simulink model "proyectoscada"  (R2016b)
settings: Solver=ode1  StartTime=0.0  StopTime=inf  FixedStep=50e-6  RelTol=1e-3
libraries: powerlib x17, rtlab x15, powerlib_meascontrol x10, sps_avr x1
settings Model: Creator=Estudiante  LastModifiedBy=Laboratorio

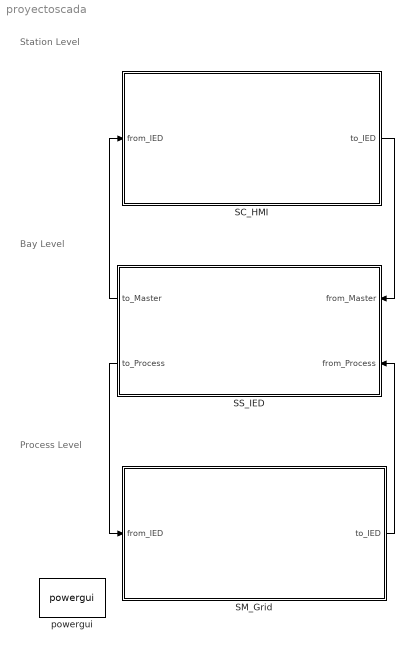
== system proyectoscada ==
  note: Station Level
  note: Bay Level
  note: Process Level
  SC_HMI : Subsystem
  SM_Grid : Subsystem
  SS_IED : Subsystem
  powergui : powerlib/powergui  Priority=1  SimulationMode=Discrete  SolverType=Backward Euler  SampleTime=50e-6  frequency=60  SPID=off  DisableSnubberDevices=off  DisableRonSwitches=off  DisableVfSwitches=off  SwTol=0  DisplayEquations=off  Interpol=off  ExternalGateDelay=off  methode=off  Ts=10  FunctionMessages=off  echomessages=off  HookPort=off  EnableUseOfTLC=off  x0status=blocks  frequencyindice=60  Pbase=100e6  ErrMax=1e-4  Iterations=50  UnitsV=kV  UnitsW=MW  buscounter=0  RestoreLinks=warning  ResistiveCurrentMeasurement=off  Frange=[0:2:500]  Ylog=off  Xlog=on  ShowGrid=off  save=off  variable=ZData  structure=0  ZoomFFT=off  StartTime=0.0  cycles=1  DisplayStyle=1  fundamental=60  FreqAxis=off  MaxFrequency=1000  frequencyindicesteady=1  RmsSteady=1  display=off
  wires:
  SS_IED/2(to_Process) -> SM_Grid/1(from_IED)
  SM_Grid/1(to_IED) -> SS_IED/2(from_Process)
  SC_HMI/1(to_IED) -> SS_IED/1(from_Master)
  SS_IED/1(to_Master) -> SC_HMI/1(from_IED)

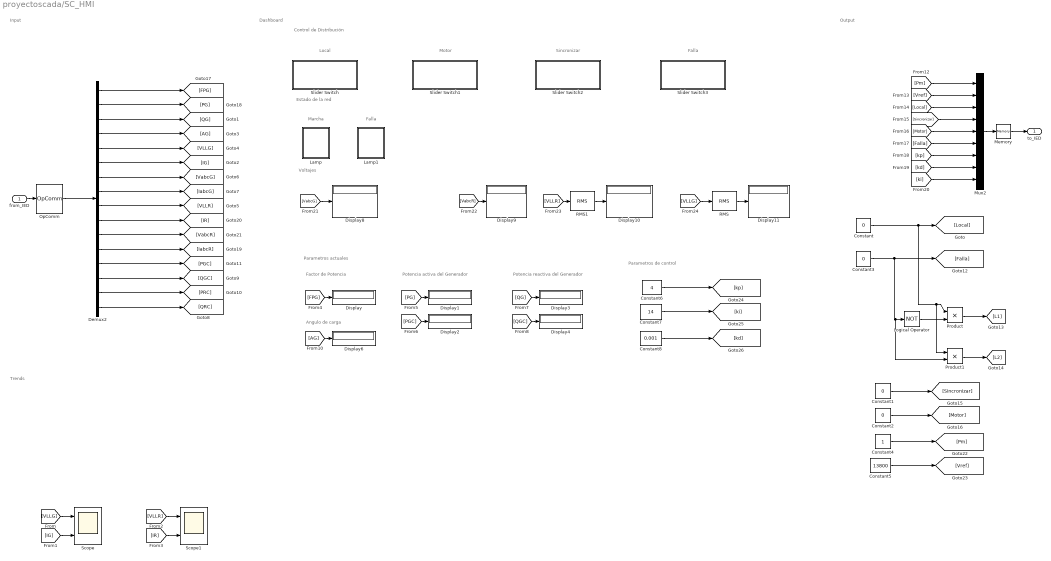
== system proyectoscada/SC_HMI ==
  note: Dashboard
  note: Input
  note: Factor de Potencia
  note: Falla
  note: Marcha
  note: Control de Distribución
  note: Falla
  note: Motor
  note: Sincronizar
  note: Local
  note: Estado de la red
  note: Voltajes
  note: Parametros actuales
  note: Potencia activa del Generador
  note: Potencia reactiva del Generador
  note: Angulo de carga
  note: Trends
  note: Output
  note: Parametros de control
  from_IED : Inport
  Constant{,1..3} (4 alike) : Constant  Value=0
  Constant4 : Constant
  Constant5 : Constant  Value=13800
  Constant6 : Constant  Value=4
  Constant7 : Constant  Value=14
  Constant8 : Constant  Value=0.001
  Demux2 : Demux  Outputs=[1 1 1 1 1 1 3 3 1 1 3 3 1 1 1 1]
  Display{,1..4,6,8..11} (10 alike) : Display
  Lamp : Subsystem  DialogController=hmiCreateDDGDialog  IsWebBlock=on  mask(MWDashboardBlock){webBlockId=f6681ff5-1f51-4868-82b0-294eaddaf335, webBlockType=lamp, ShowInLibBrowser=on, ShowInitialText=on, HMISrcModelName=proyectoscada}
      mask prompts: webBlockType "WebBlock Type"; HMISrcModelName "Source Model"
      mask help: SimulinkHMI:dialogs:LampDialogDesc
      mask Help: helpview([docroot '/mapfiles/simulink.map'], 'hmi_lamp')
      mask Display:
      | if strcmp(get_param(bdroot(gcb),'BlockDiagramType'), 'library')
      |     image([(matlabroot) '/toolbox/simulink/hmi/icons/Lamp.png']);
      | end
  Lamp1 : Subsystem  DialogController=hmiCreateDDGDialog  IsWebBlock=on  mask(MWDashboardBlock){webBlockId=feaf209c-0dec-4196-b8e9-5f0cb4ab0a6e, webBlockType=lamp, ShowInLibBrowser=on, ShowInitialText=on, HMISrcModelName=proyectoscada}
      mask prompts: webBlockType "WebBlock Type"; HMISrcModelName "Source Model"
      mask help: SimulinkHMI:dialogs:LampDialogDesc
      mask Help: helpview([docroot '/mapfiles/simulink.map'], 'hmi_lamp')
      mask Display:
      | if strcmp(get_param(bdroot(gcb),'BlockDiagramType'), 'library')
      |     image([(matlabroot) '/toolbox/simulink/hmi/icons/Lamp.png']);
      | end
  Logical Operator : Logic  Operator=NOT  AllPortsSameDT=off  OutDataTypeStr=boolean
  Memory : Memory
  Mux2 : Mux  Inputs=9
  OpComm : rtlab/OpComm  nbport=1  groupe_acq=1  subsys_rate=0  st=0  Synchronization=on  Interpolation=on  Threshold=1.0  Missed_Data=off  Sim_Time=off  Samples=off  dynSigOut=off  from_console=0  warning_done=off  writeOpCommFile=off  Offset=off
  Product : Product
  Product1 : Product
  RMS : powerlib_meascontrol/Measurements/RMS  TrueRMS=on  Freq=60  RMSInit=120  Ts=0
  RMS1 : powerlib_meascontrol/Measurements/RMS  TrueRMS=on  Freq=60  RMSInit=120  Ts=0
  Scope : Scope  NumInputPorts=2
  Scope1 : Scope  NumInputPorts=2
  Slider Switch : Subsystem  DialogController=hmiCreateDDGDialog  IsWebBlock=on  mask(MWDashboardBlock){webBlockId=af04694c-61e9-4dac-be57-759f0575d0dc, webBlockType=sliderswitch, ShowInLibBrowser=on, ShowInitialText=on, HMISrcModelName=proyectoscada}
      mask prompts: webBlockId "WebBlock Id"; webBlockType "WebBlock Type"; HMISrcModelName "Source Model"
      mask help: SimulinkHMI:dialogs:SwitchDialogDesc
      mask Help: helpview([docroot '/mapfiles/simulink.map'], 'hmi_slider_switch')
      mask Display:
      | if strcmp(get_param(bdroot(gcb),'BlockDiagramType'), 'library')
      |     image([(matlabroot) '/toolbox/simulink/hmi/icons/SliderSwitch.png']);
      | end
  Slider Switch1 : Subsystem  DialogController=hmiCreateDDGDialog  IsWebBlock=on  mask(MWDashboardBlock){webBlockId=260ccb06-39bd-439d-99f7-5433d5649649, webBlockType=sliderswitch, ShowInLibBrowser=on, ShowInitialText=on, HMISrcModelName=proyectoscada}
      mask prompts: webBlockId "WebBlock Id"; webBlockType "WebBlock Type"; HMISrcModelName "Source Model"
      mask help: SimulinkHMI:dialogs:SwitchDialogDesc
      mask Help: helpview([docroot '/mapfiles/simulink.map'], 'hmi_slider_switch')
      mask Display:
      | if strcmp(get_param(bdroot(gcb),'BlockDiagramType'), 'library')
      |     image([(matlabroot) '/toolbox/simulink/hmi/icons/SliderSwitch.png']);
      | end
  Slider Switch2 : Subsystem  DialogController=hmiCreateDDGDialog  IsWebBlock=on  mask(MWDashboardBlock){webBlockId=4ed2cfc3-4726-40f0-a434-b0a17b732f1d, webBlockType=sliderswitch, ShowInLibBrowser=on, ShowInitialText=on, HMISrcModelName=proyectoscada}
      mask prompts: webBlockId "WebBlock Id"; webBlockType "WebBlock Type"; HMISrcModelName "Source Model"
      mask help: SimulinkHMI:dialogs:SwitchDialogDesc
      mask Help: helpview([docroot '/mapfiles/simulink.map'], 'hmi_slider_switch')
      mask Display:
      | if strcmp(get_param(bdroot(gcb),'BlockDiagramType'), 'library')
      |     image([(matlabroot) '/toolbox/simulink/hmi/icons/SliderSwitch.png']);
      | end
  Slider Switch3 : Subsystem  DialogController=hmiCreateDDGDialog  IsWebBlock=on  mask(MWDashboardBlock){webBlockId=741865aa-7a89-4127-9b99-651b078b7427, webBlockType=sliderswitch, ShowInLibBrowser=on, ShowInitialText=on, HMISrcModelName=proyectoscada}
      mask prompts: webBlockId "WebBlock Id"; webBlockType "WebBlock Type"; HMISrcModelName "Source Model"
      mask help: SimulinkHMI:dialogs:SwitchDialogDesc
      mask Help: helpview([docroot '/mapfiles/simulink.map'], 'hmi_slider_switch')
      mask Display:
      | if strcmp(get_param(bdroot(gcb),'BlockDiagramType'), 'library')
      |     image([(matlabroot) '/toolbox/simulink/hmi/icons/SliderSwitch.png']);
      | end
  to_IED : Outport
  wires:
  [FPG] -> Display/1
  Constant6/1 -> [kp]
  Constant3/1 -> [Falla], Product1/2, Logical Operator/1
  Demux2/4 -> [AG]
  Demux2/8 -> [IabcG]
  Demux2/3 -> [QG]
  Demux2/11 -> [VabcR]
  Demux2/12 -> [IabcR]
  Demux2/5 -> [VLLG]
  Demux2/6 -> [IG]
  Demux2/9 -> [VLLR]
  Demux2/10 -> [IR]
  Demux2/2 -> [PG]
  Demux2/7 -> [VabcG]
  Demux2/1 -> [FPG]
  Product1/1 -> [L2]
  Logical Operator/1 -> Product/2
  Demux2/15 -> [PRC]
  Demux2/16 -> [QRC]
  Demux2/14 -> [QGC]
  Demux2/13 -> [PGC]
  Constant8/1 -> [kd]
  [Local] -> Mux2/3
  [ki] -> Mux2/9
  [Motor] -> Mux2/5
  [Vref] -> Mux2/2
  [Pm] -> Mux2/1
  [kd] -> Mux2/8
  [Sincronizar] -> Mux2/4
  [Falla] -> Mux2/6
  [kp] -> Mux2/7
  Constant1/1 -> [Sincronizar]
  [AG] -> Display6/1
  Constant2/1 -> [Motor]
  [PG] -> Display1/1
  Product/1 -> [L1]
  Constant4/1 -> [Pm]
  Constant5/1 -> [Vref]
  Constant7/1 -> [ki]
  [IG] -> Scope/2
  [QG] -> Display3/1
  [QGC] -> Display4/1
  [VLLR] -> Scope1/1
  [PGC] -> Display2/1
  [IR] -> Scope1/2
  [VLLG] -> Scope/1
  Constant/1 -> Product1/1, Product/1, [Local]
  [VabcG] -> Display8/1
  [VabcR] -> Display9/1
  [VLLG] -> RMS/1
  RMS/1 -> Display11/1
  [VLLR] -> RMS1/1
  RMS1/1 -> Display10/1
  Mux2/1 -> Memory/1
  Memory/1 -> to_IED/1
  from_IED/1 -> OpComm/1
  OpComm/1 -> Demux2/1

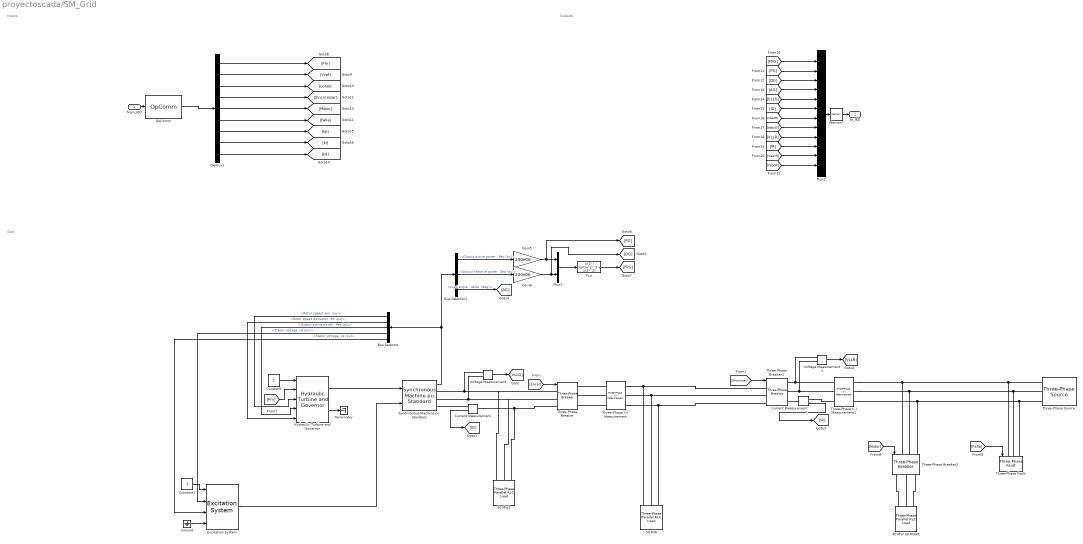
== system proyectoscada/SM_Grid ==
  note: Inputs
  note: Grid
  note: Outputs
  from_IED : Inport
  40 MW 30 MVAR : powerlib/Elements/Three-Phase Parallel RLC Load  LConnTagsString=A|B|C  Configuration=Y (grounded)  NominalVoltage=13800  Vabc=[1e3 1e3 1e3]  Vabcp=[1e3 1e3 1e3]  NominalFrequency=60  UnbalancedPower=off  ActivePower=40e6  InductivePower=30e6  CapacitivePower=0  Pabc=[10e3 9e3 11e3]  QLabc=[100 90 110]  QCabc=[100 90 110]  Pabcp=[10e3 9e3 11e3]  QLabcp=[100 90 110]  QCabcp=[100 90 110]  Measurements=None  LoadType=constant Z
  50 MW : powerlib/Elements/Three-Phase Parallel RLC Load  LConnTagsString=A|B|C  Configuration=Y (grounded)  NominalVoltage=13800  Vabc=[1e3 1e3 1e3]  Vabcp=[1e3 1e3 1e3]  NominalFrequency=60  UnbalancedPower=off  ActivePower=50e6  InductivePower=0  CapacitivePower=0  Pabc=[10e3 9e3 11e3]  QLabc=[100 90 110]  QCabc=[100 90 110]  Pabcp=[10e3 9e3 11e3]  QLabcp=[100 90 110]  QCabcp=[100 90 110]  Measurements=None  LoadType=constant Z
  50 MW1 : powerlib/Elements/Three-Phase Parallel RLC Load  LConnTagsString=A|B|C  Configuration=Y (grounded)  NominalVoltage=13800  Vabc=[1e3 1e3 1e3]  Vabcp=[1e3 1e3 1e3]  NominalFrequency=60  UnbalancedPower=off  ActivePower=50e6  InductivePower=0  CapacitivePower=0  Pabc=[10e3 9e3 11e3]  QLabc=[100 90 110]  QCabc=[100 90 110]  Pabcp=[10e3 9e3 11e3]  QLabcp=[100 90 110]  QCabcp=[100 90 110]  Measurements=None  LoadType=constant Z
  Bus Selector : BusSelector  OutputSignals="Mechanical.Rotor speed  wm  (pu),Mechanical.Rotor speed deviation  dw (pu),Output active power   Peo (pu),dq0 components.Stator voltage  vd (pu),dq0 components.Stator voltage  vq (pu)"
  Bus Selector1 : BusSelector  OutputSignals="Output active power   Peo (pu),Output reactive power  Qeo (pu),Load angle   delta  (deg)"
  Constant : Constant
  Constant1 : Constant
  Current Measurement : powerlib/Measurements/Current Measurement  PhasorSimulation=off  OutputType=Complex  PSBequivalent=0
  Current Measurement1 : powerlib/Measurements/Current Measurement  PhasorSimulation=off  OutputType=Complex  PSBequivalent=0
  Demux1 : Demux  Outputs=9
  Excitation System : sps_avr/Excitation System  tr=20e-3  reg=[ 300, 0.001 ]  exc=[ 1, 0 ]  tgr=[ 0, 0 ]  damp=[ 0.001, 0.1 ]  sat=[ 0, 0 ]  lim=[ -11.5, 11.5, 0 ]  v0="[1.0  1.28]"
  Fcn : Fcn  Expr=u(1) / sqrt(u(1)^2 + u(2)^2)
  Gain5 : Gain  Gain=200e06
  Gain6 : Gain  Gain=200e06
  Ground : Ground
  Hydraulic Turbine and Governor : powerlib/Machines/Hydraulic Turbine and Governor  sm="[ 10/3  0.07 ]"  gate="[  0.01  0.97518  -0.1  0.1 ]"  reg="[  0.05  1.163  0.105  0  0.01  ]"  hyd="[  0  2.67  ]"  dref=0  po=0.7516
  Memory : Memory
  Mux1 : Mux  Inputs=2
  Mux2 : Mux  Inputs=12
  OpComm : rtlab/OpComm  nbport=1  groupe_acq=1  subsys_rate=0  st=0  Synchronization=on  Interpolation=on  Threshold=1.0  Missed_Data=off  Sim_Time=off  Samples=off  dynSigOut=off  from_console=0  warning_done=off  writeOpCommFile=off  Offset=off
  Synchronous Machine pu Standard : powerlib/Machines/Synchronous Machine pu Standard  PresetModel=No  MechanicalLoad=Mechanical power Pm  ShowDetailedParameters=on  RotorType=Salient-pole  Units=per unit standard parameters  MeasurementBus=off  NominalParameters=[200E06 13800 60]  Reactances1=[ 1.81, 0.3, 0.23, 1.76, 0.65, 0.25, 0.15 ]  Reactances2=[1.305 0.296 0.252 0.474 0.243 0.18]  dAxisTimeConstants=Short-circuit  qAxisTimeConstants=Open-circuit  TimeConstants1="[ 4.4849  0.0681  0.1  ]"  TimeConstants2=[ 8.0, 0.03, 1.0, 0.07 ]  TimeConstants3="[  4.49  0.0681  0.0513  ]"  TimeConstants4=[ 8.0, 0.03, 0.3371, 0.0295 ]  TimeConstants5=[ 1.01, 0.053, 0.1 ]  TimeConstants6=[ 1.3201, 0.023, 1.0, 0.07 ]  TimeConstants7=[0.012 0.003 0.003]  TimeConstants8=[ 1.3201, 0.0231, 0.3371, 0.0295 ]  StatorResistance=2.8544e-3  Mechanical=[3.2 0 2]  PolePairs=20  InitialConditions="[ 0  -94.2826  0.75018 0.75018 0.75018  -24.943  -144.943  95.057  1.2907   ]"  SetSaturation=off  Saturation=[0.6404,0.7127,0.8441,0.9214,0.9956,1.082,1.19,1.316,1.457;0.7,0.7698,0.8872,0.9466,0.9969,1.046,1.1,1.151,1.201]  LoadFlowParameters=[1 150000000 0 0 0]  TsPowergui=0  TsBlock=50e-6  IterativeModel=Trapezoidal non iterative  IterativeDiscreteModel=Trapezoidal iterative (alg. loop)  BusType=PV  Pref=150000000  Qref=0  Qmin=-inf  Qmax=inf  PLF=0  QLF=0
  Terminator : Terminator
  Three-Phase V-I Measurement : powerlib/Measurements/Three-Phase V-I Measurement  VoltageMeasurement=phase-to-ground  SetLabelV=on  LabelV=VabcG  Vpu=off  VpuLL=off  CurrentMeasurement=yes  SetLabelI=on  LabelI=IabcG  Ipu=off  Pbase=100e6  Vbase=500e3  OutputType=Complex  PhasorSimulation=off  PSBequivalent=0
  Three-Phase V-I Measurement1 : powerlib/Measurements/Three-Phase V-I Measurement  VoltageMeasurement=phase-to-ground  SetLabelV=on  LabelV=VabcR  Vpu=off  VpuLL=off  CurrentMeasurement=yes  SetLabelI=on  LabelI=IabcR  Ipu=off  Pbase=100e6  Vbase=500e3  OutputType=Complex  PhasorSimulation=off  PSBequivalent=0
  Three-Phase Breaker : powerlib/Elements/Three-Phase Breaker  InitialState=open  SwitchA=on  SwitchB=on  SwitchC=on  SwitchTimes="[1/60  5/60]"  External=on  BreakerResistance=0.01  SnubberResistance=1e6  SnubberCapacitance=inf  Measurements=None
  Three-Phase Breaker1 : powerlib/Elements/Three-Phase Breaker  InitialState=open  SwitchA=on  SwitchB=on  SwitchC=on  SwitchTimes="[1/60  5/60]"  External=on  BreakerResistance=0.01  SnubberResistance=1e6  SnubberCapacitance=inf  Measurements=None
  Three-Phase Breaker2 : powerlib/Elements/Three-Phase Breaker  InitialState=open  SwitchA=on  SwitchB=on  SwitchC=on  SwitchTimes="[1/60  5/60]"  External=on  BreakerResistance=0.01  SnubberResistance=1e6  SnubberCapacitance=inf  Measurements=None
  Three-Phase Fault : powerlib/Elements/Three-Phase Fault  InitialStates=0  FaultA=on  FaultB=on  FaultC=on  GroundFault=on  SwitchTimes="[1/60  5/60]"  External=on  SwitchStatus=NaN  FaultResistance=0.001  GroundResistance=0.01  SnubberResistance=1e6  SnubberCapacitance=inf  Measurements=None
  Three-Phase Source : powerlib/Electrical Sources/Three-Phase Source  InternalConnection=Yg  VoltagePhases=off  Voltage=13800  PhaseAngle=5  Voltage_phases=[25e3 25e3 25e3]/sqrt(3)  PhaseAngles_phases=[0 -120 +120]  Frequency=60  NonIdealSource=on  SpecifyImpedance=on  Resistance=0.8929  Inductance=16.58e-3  ShortCircuitLevel=400e6  BaseVoltage=13800  XRratio=10  BusType=swing  Pref=10e3  Qref=0  Prefabc=[10e3, 10e3, 10e3]  Qrefabc=[0, 0, 0]  Qmin=-inf  Qmax=inf
  Voltage Measurement : powerlib/Measurements/Voltage Measurement  PhasorSimulation=off  OutputType=Complex  PSBequivalent=0
  Voltage Measurement1 : powerlib/Measurements/Voltage Measurement  PhasorSimulation=off  OutputType=Complex  PSBequivalent=0
  to_IED : Outport
  wires:
  Voltage Measurement/1 -> [VLLG]
  Current Measurement/1 -> [IG]
  Voltage Measurement1/1 -> [VLLR]
  [Falla] -> Three-Phase Fault/1
  Current Measurement1/1 -> [IR]
  Demux1/3 -> [Local]
  [VLLR] -> Mux2/9
  [VabcR] -> Mux2/11
  [PG] -> Mux2/2
  [IabcG] -> Mux2/8
  [VabcG] -> Mux2/7
  [AG] -> Mux2/4
  [VLLG] -> Mux2/5
  Bus Selector1/3 -> [AG]  "<Load angle   delta  (deg)>"
  Bus Selector1/1 -> Gain5/1  "<Output active power   Peo (pu)>"
  Mux1/1 -> Fcn/1
  Bus Selector1/2 -> Gain6/1  "<Output reactive power  Qeo (pu)>"
  Fcn/1 -> [FPG]
  [FPG] -> Mux2/1
  Demux1/9 -> [kd]
  Demux1/7 -> [kp]
  Demux1/6 -> [Falla]
  Demux1/5 -> [Motor]
  Demux1/1 -> [Pm]
  Demux1/2 -> [Vref]
  [IR] -> Mux2/10
  [IabcR] -> Mux2/12
  [QG] -> Mux2/3
  Demux1/4 -> [Sincronizar]
  [IG] -> Mux2/6
  Demux1/8 -> [ki]
  Hydraulic Turbine and Governor/1 -> Synchronous Machine pu Standard/1
  Hydraulic Turbine and Governor/2 -> Terminator/1
  Constant/1 -> Hydraulic Turbine and Governor/1
  Bus Selector/3 -> Hydraulic Turbine and Governor/4  "<Output active power   Peo (pu)>"
  Bus Selector/1 -> Hydraulic Turbine and Governor/3  "<Rotor speed  wm  (pu)>"
  Bus Selector/2 -> Hydraulic Turbine and Governor/5  "<Rotor speed deviation  dw (pu)>"
  Synchronous Machine pu Standard/1 -> Bus Selector1/1, Bus Selector/1
  [Pm] -> Hydraulic Turbine and Governor/2
  [Local] -> Three-Phase Breaker/1
  [Sincronizar] -> Three-Phase Breaker1/1
  Gain5/1 -> [PG], Mux1/1
  Gain6/1 -> [QG], Mux1/2
  ? -> ?
  [Motor] -> Three-Phase Breaker2/1
  Mux2/1 -> Memory/1
  Memory/1 -> to_IED/1
  from_IED/1 -> OpComm/1
  OpComm/1 -> Demux1/1
  Constant1/1 -> Excitation System/1
  Bus Selector/4 -> Excitation System/2  "<Stator voltage  vd (pu)>"
  Bus Selector/5 -> Excitation System/3  "<Stator voltage  vq (pu)>"
  Ground/1 -> Excitation System/4
  Excitation System/1 -> Synchronous Machine pu Standard/2
  connections:
  Current Measurement1/LConn1 -- Three-Phase Breaker1/RConn3
  Three-Phase V-I Measurement/LConn1 -- Three-Phase Breaker/RConn1
  Voltage Measurement/LConn2 -- 50 MW1/LConn2 -- Three-Phase Breaker/LConn2 -- Synchronous Machine pu Standard/RConn2
  Three-Phase V-I Measurement/LConn3 -- Three-Phase Breaker/RConn3
  Three-Phase V-I Measurement1/LConn1 -- Voltage Measurement1/LConn1 -- Three-Phase Breaker1/RConn1
  Voltage Measurement/LConn1 -- 50 MW1/LConn1 -- Three-Phase Breaker/LConn1 -- Synchronous Machine pu Standard/RConn1
  Three-Phase V-I Measurement1/RConn1 -- Three-Phase Breaker2/LConn1 -- Three-Phase Fault/LConn1 -- Three-Phase Source/RConn1
  Three-Phase V-I Measurement1/RConn2 -- Three-Phase Breaker2/LConn2 -- Three-Phase Fault/LConn2 -- Three-Phase Source/RConn2
  Three-Phase V-I Measurement/LConn2 -- Three-Phase Breaker/RConn2
  Current Measurement1/RConn1 -- Three-Phase V-I Measurement1/LConn3
  Three-Phase V-I Measurement1/LConn2 -- Voltage Measurement1/LConn2 -- Three-Phase Breaker1/RConn2
  Three-Phase V-I Measurement/RConn3 -- Three-Phase Breaker1/LConn3 -- 50 MW/LConn3
  Three-Phase Breaker1/LConn2 -- 50 MW/LConn2 -- Three-Phase V-I Measurement/RConn2
  Three-Phase V-I Measurement1/RConn3 -- Three-Phase Breaker2/LConn3 -- Three-Phase Fault/LConn3 -- Three-Phase Source/RConn3
  Current Measurement/RConn1 -- Synchronous Machine pu Standard/RConn3
  Three-Phase V-I Measurement/RConn1 -- Three-Phase Breaker1/LConn1 -- 50 MW/LConn1
  Current Measurement/LConn1 -- 50 MW1/LConn3 -- Three-Phase Breaker/LConn3
  40 MW 30 MVAR/LConn2 -- Three-Phase Breaker2/RConn2
  40 MW 30 MVAR/LConn1 -- Three-Phase Breaker2/RConn1
  40 MW 30 MVAR/LConn3 -- Three-Phase Breaker2/RConn3

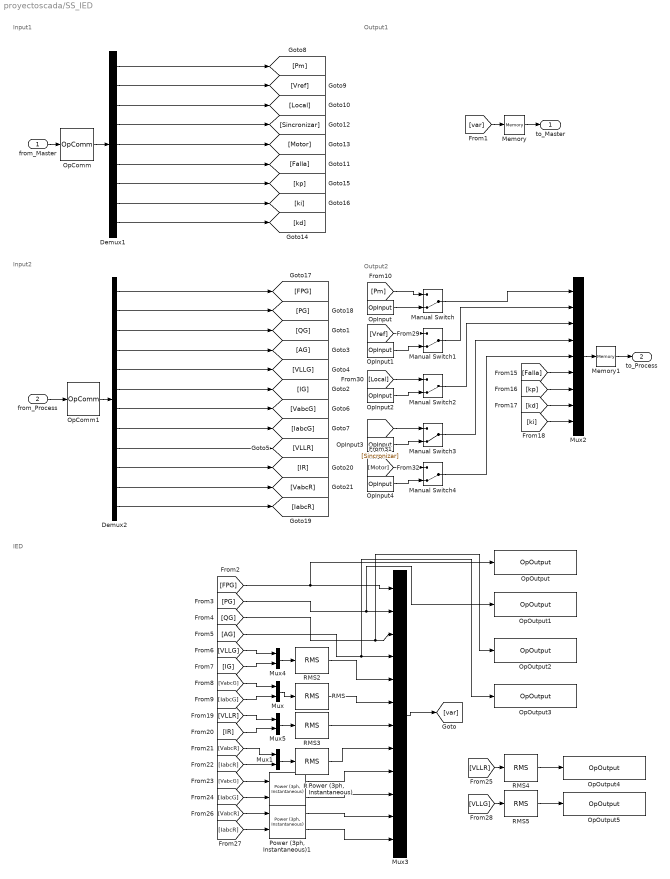
== system proyectoscada/SS_IED ==
  note: IED
  note: Output2
  note: Input2
  note: Output1
  note: Input1
  from_Master : Inport
  from_Process : Inport  Port=2
  Demux1 : Demux  Outputs=9
  Demux2 : Demux  Outputs=[1 1 1 1 1 1 3 3 1 1 3 3]
  Manual Switch{,1..4} (5 alike) : ManualSwitch  CurrentSetting=0
  Memory : Memory
  Memory1 : Memory
  Mux{,1,4..5} (4 alike) : Mux  Inputs=2
  Mux2 : Mux  Inputs=9
  Mux3 : Mux  Inputs=12
  OpComm : rtlab/OpComm  nbport=1  groupe_acq=1  subsys_rate=0  st=0  Synchronization=on  Interpolation=on  Threshold=1.0  Missed_Data=off  Sim_Time=off  Samples=off  dynSigOut=off  from_console=1  warning_done=off  writeOpCommFile=off  Offset=off
  OpComm1 : rtlab/OpComm  nbport=1  groupe_acq=1  subsys_rate=0  st=0  Synchronization=on  Interpolation=on  Threshold=1.0  Missed_Data=off  Sim_Time=off  Samples=off  dynSigOut=off  from_console=0  warning_done=off  writeOpCommFile=off  Offset=off
  OpInput : rtlab/OpInput  identifier_use=Pm  identifier_hide=Pm  nb_parents_identifier=0  passthrough=off  init_value=0  value_type=double  create_alias=on
  OpInput1 : rtlab/OpInput  identifier_use=Vref  identifier_hide=Vref  nb_parents_identifier=0  passthrough=off  init_value=0  value_type=double  create_alias=on
  OpInput2 : rtlab/OpInput  identifier_use=Local  identifier_hide=Local  nb_parents_identifier=0  passthrough=off  init_value=0  value_type=double  create_alias=on
  OpInput3 : rtlab/OpInput  identifier_use=Sincronizar  identifier_hide=Sincronizar  nb_parents_identifier=0  passthrough=off  init_value=0  value_type=double  create_alias=on
  OpInput4 : rtlab/OpInput  identifier_use=Motor  identifier_hide=Motor  nb_parents_identifier=0  passthrough=off  init_value=0  value_type=double  create_alias=on
  OpOutput : rtlab/OpOutput  identifier_use=FPG  identifier_hide=FPG  nb_parents_identifier=0
  OpOutput1 : rtlab/OpOutput  identifier_use=PG  identifier_hide=PG  nb_parents_identifier=0
  OpOutput2 : rtlab/OpOutput  identifier_use=QG  identifier_hide=QG  nb_parents_identifier=0
  OpOutput3 : rtlab/OpOutput  identifier_use=AG  identifier_hide=AG  nb_parents_identifier=0
  OpOutput4 : rtlab/OpOutput  identifier_use=VLLR  identifier_hide=VLLR  nb_parents_identifier=0
  OpOutput5 : rtlab/OpOutput  identifier_use=VLLG  identifier_hide=VLLG  nb_parents_identifier=0
  "Power (3ph, Instantaneous)" : powerlib_meascontrol/Measurements/Power (3ph, Instantaneous)
  "Power (3ph, Instantaneous)1" : powerlib_meascontrol/Measurements/Power (3ph, Instantaneous)
  RMS{,1..5} (6 alike) : powerlib_meascontrol/Measurements/RMS  TrueRMS=on  Freq=60  RMSInit=120  Ts=0
  to_Master : Outport
  to_Process : Outport  Port=2
  wires:
  Demux2/7 -> [VabcG]
  Demux2/6 -> [IG]
  Demux2/5 -> [VLLG]
  Demux2/2 -> [PG]
  Demux2/8 -> [IabcG]
  Demux2/9 -> [VLLR]
  Demux2/1 -> [FPG]
  Demux2/4 -> [AG]
  Demux2/3 -> [QG]
  Demux2/12 -> [IabcR]
  Mux3/1 -> [var]
  Demux2/10 -> [IR]
  Demux1/9 -> [kd]
  Demux1/7 -> [kp]
  Demux1/6 -> [Falla]
  Demux1/3 -> [Local]
  Demux1/8 -> [ki]
  Demux1/5 -> [Motor]
  Demux1/4 -> [Sincronizar]
  Demux1/2 -> [Vref]
  Demux1/1 -> [Pm]
  Demux2/11 -> [VabcR]
  [IabcG] -> "Power (3ph, Instantaneous)"/2
  [VabcR] -> "Power (3ph, Instantaneous)1"/1
  [IabcR] -> "Power (3ph, Instantaneous)1"/2
  [VabcG] -> "Power (3ph, Instantaneous)"/1
  [FPG] -> OpOutput/1, Mux3/1
  [PG] -> OpOutput1/1, Mux3/2
  [QG] -> OpOutput2/1, Mux3/3
  [AG] -> OpOutput3/1, Mux3/4
  Mux/1 -> RMS/1
  [VabcG] -> Mux/1
  [IabcG] -> Mux/2
  Mux4/1 -> RMS2/1
  [VLLG] -> Mux4/1
  [IG] -> Mux4/2
  RMS2/1 -> Mux3/5
  RMS/1 -> Mux3/6
  Mux1/1 -> RMS1/1
  [VabcR] -> Mux1/1
  [IabcR] -> Mux1/2
  Mux5/1 -> RMS3/1
  [VLLR] -> Mux5/1
  [IR] -> Mux5/2
  RMS3/1 -> Mux3/7
  RMS1/1 -> Mux3/8
  "Power (3ph, Instantaneous)"/1 -> Mux3/9
  "Power (3ph, Instantaneous)"/2 -> Mux3/10
  "Power (3ph, Instantaneous)1"/1 -> Mux3/11
  "Power (3ph, Instantaneous)1"/2 -> Mux3/12
  [var] -> Memory/1
  Memory/1 -> to_Master/1
  Mux2/1 -> Memory1/1
  Memory1/1 -> to_Process/1
  from_Master/1 -> OpComm/1
  OpComm/1 -> Demux1/1
  OpComm1/1 -> Demux2/1
  from_Process/1 -> OpComm1/1
  [VLLR] -> RMS4/1
  [VLLG] -> RMS5/1
  RMS4/1 -> OpOutput4/1
  RMS5/1 -> OpOutput5/1
  OpInput/1 -> Manual Switch/2
  [Pm] -> Manual Switch/1
  Manual Switch/1 -> Mux2/1
  [Vref] -> Manual Switch1/1
  OpInput1/1 -> Manual Switch1/2
  OpInput2/1 -> Manual Switch2/2
  [Local] -> Manual Switch2/1
  OpInput3/1 -> Manual Switch3/2
  [Sincronizar] -> Manual Switch3/1
  OpInput4/1 -> Manual Switch4/2
  [Motor] -> Manual Switch4/1
  Manual Switch1/1 -> Mux2/2
  Manual Switch2/1 -> Mux2/3
  Manual Switch3/1 -> Mux2/4
  Manual Switch4/1 -> Mux2/5
  [ki] -> Mux2/9
  [kd] -> Mux2/8
  [kp] -> Mux2/7
  [Falla] -> Mux2/6

== system proyectoscada/SC_HMI/Lamp ==

== system proyectoscada/SC_HMI/Lamp1 ==

== system proyectoscada/SC_HMI/Slider Switch ==

== system proyectoscada/SC_HMI/Slider Switch1 ==

== system proyectoscada/SC_HMI/Slider Switch2 ==

== system proyectoscada/SC_HMI/Slider Switch3 ==
